simulink model "raspberrypi_MQTT_final"  (R2022b)
settings: Solver=FixedStepAuto  StartTime=0.0  StopTime=inf  RelTol=1e-3  EnableMultiTasking=on
undefined symbols (not defined in the file): hw
libraries: raspberrypiAVlib x1, raspberrypiIOTlib x1, dspspect3 x1, audiofilters x1, dspsigops x1
settings Model: Creator=The MathWorks, Inc.  LastModifiedBy=alex
settings SolverCC: AlgebraicLoopSolver=TrustRegion  PositivePriorityOrder=on  MaxZcPerStep=1
settings DataIOCC: ReturnWorkspaceOutputs=off
settings OptimizationCC: EnhancedBackFolding=on  PassReuseOutputArgsThreshold=0  MaxStackSize=64  OptimizeBlockOrder=speed  DifferentSizesBufferReuse=on  OptimizationCustomize=off
settings DebuggingCC: ParameterTunabilityLossMsg=error  UnconnectedInputMsg=warning  UnconnectedOutputMsg=warning  UnconnectedLineMsg=warning  PregeneratedLibrarySubsystemCodeDiagnostic=none  SFMachineParentedDataDiag=warning  ArithmeticOperatorsInVariantConditions=warning
settings HardwareCC: ProdBitPerPointer=32  ProdBitPerSizeT=32  ProdBitPerPtrDiffT=32  ProdLargestAtomicInteger=Long  ProdLargestAtomicFloat=Double  ProdWordSize=32  ProdHWDeviceType=ARM Compatible->ARM Cortex  UseEmbeddedCoderFeatures=off  UseSimulinkCoderFeatures=off
settings ModelReferenceCC: EnableRefExpFcnMdlSchedulingChecks=on
settings SFSimCC: SimUseLocalCustomCode=off  MATLABDynamicMemAlloc=off  CustomCodeUndefinedFunction=UseInterfaceOnly
settings RTWCC: Description=Embedded Coder  SystemTargetFile=ert.tlc  HardwareBoard=Raspberry Pi  TLCOptions="-aInlineSetEventsForThisBaseRateFcn=TLC_FALSE -aSuppressMultiTaskScheduler=TLC_FALSE  -aRateBasedStepFcn=0"  TemplateMakefile=ert_default_tmf  GenerateReport=on  RTWUseLocalCustomCode=off  Toolchain=GNU GCC Embedded Linux  BuildConfiguration=Faster Runs  LaunchReport=on  DLArmComputeVersion=19.05
settings CodeAppCC: ForceParamTrailComments=on  OperatorAnnotations=on
settings ERTTargetCC: ERTCustomFileBanners=off  SupportContinuousTime=on  SupportNonInlinedSFcns=on  RemoveResetFunc=off  SupportVariableSizeSignals=on  ModelStepFunctionPrototypeControlCompliant=off

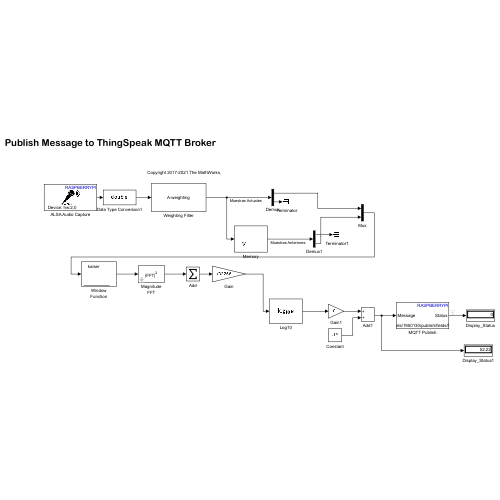
[thumbnail: Simulink's stored preview of the top-level diagram]
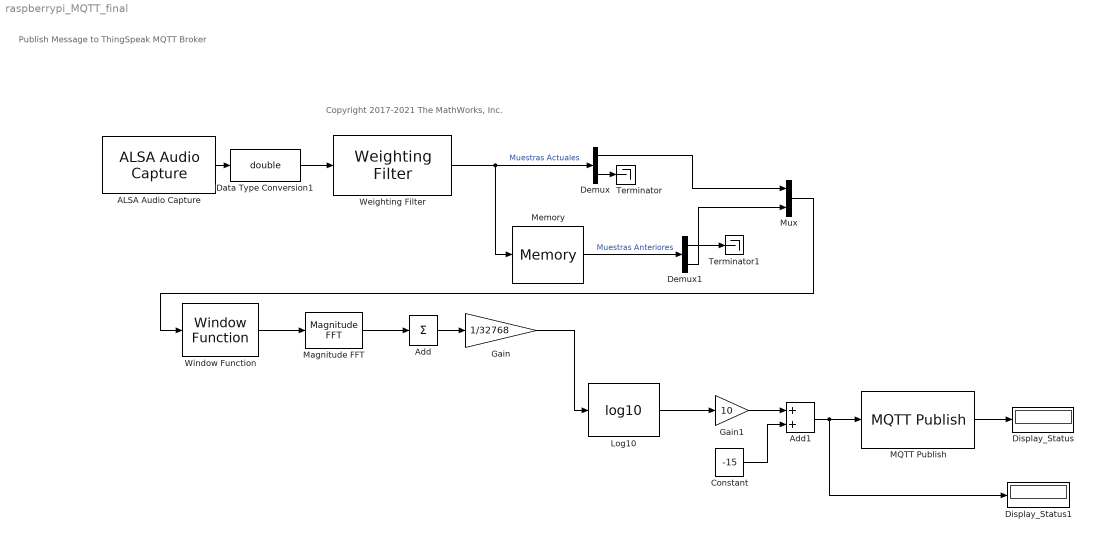
== system raspberrypi_MQTT_final ==
  note: Publish Message to ThingSpeak MQTT Broker
  note: Copyright 2017-2021 The MathWorks, Inc.
  ALSA Audio Capture : raspberrypiAVlib/ALSA Audio Capture  deviceStr=hw:2,0  DataBitDepth=16-bit integer  numberOfChannels=1  sampleRateEnum=44100  frameSize=22050  QueueDuration=0.5  blockPlatform=RASPBERRYPI
  Add : Sum  Inputs=+
  Add1 : Sum
  Constant : Constant  Value=-15
  Data Type Conversion1 : DataTypeConversion  OutDataTypeStr=double  RndMeth=Nearest
  Demux : Demux  Outputs=2
  Demux1 : Demux  Outputs=2
  Display_Status : Display
  Display_Status1 : Display
  Gain : Gain  Gain=1/32768
  Gain1 : Gain  Gain=10
  Log10 : Math  Operator=log10
  MQTT Publish : raspberrypiIOTlib/MQTT Publish  Topic=channels/1950130/publish/fields/field1  QoS=0  RetainMsg=off  blockPlatform=RASPBERRYPI
  Magnitude FFT : dspspect3/Magnitude FFT  mag_or_magsq=Magnitude squared  FFTImplementation=Auto  fftLenInherit=off  fftsize=32768  WrapInput=on
  Memory : Memory
  Mux : Mux  Inputs=2
  Terminator : Terminator
  Terminator1 : Terminator
  Weighting Filter : audiofilters/Weighting Filter  Method=A-weighting  InheritSampleRate=off  SampleRate=44100  SimulateUsing=Code generation  WorkspaceVariableName=myFilt  OverwriteExportVariable=on  MaskClassType=No mask
  Window Function : dspsigops/Window Function  winmode=Apply window to input  wintype=Kaiser  sampmode=Continuous  samptime=1  N=64  Rs=50  beta=5  winsamp=Symmetric  UserWindow=hamming  OptParams=off  UserParams={'symmetric'}  dataType=double  isSigned=on  wordLen=16  udDataType=sfix(16)  fracBitsMode=Best precision  numFracBits=15  roundingMode=Floor  overflowMode=off  numSidelobes=4  sidelobeLevel=-30
  wires:
  Data Type Conversion1/1 -> Weighting Filter/1
  Log10/1 -> Gain1/1
  Add/1 -> Gain/1
  Gain/1 -> Log10/1
  Magnitude FFT/1 -> Add/1
  Demux1/2 -> Mux/2
  Demux/2 -> Terminator/1
  Memory/1 -> Demux1/1  "Muestras Anteriores"
  Weighting Filter/1 -> Demux/1, Memory/1  "Muestras Actuales"
  Demux1/1 -> Terminator1/1
  Window Function/1 -> Magnitude FFT/1
  Constant/1 -> Add1/2
  Mux/1 -> Window Function/1
  Gain1/1 -> Add1/1
  Demux/1 -> Mux/1
  Add1/1 -> Display_Status1/1, MQTT Publish/1
  MQTT Publish/1 -> Display_Status/1
  ALSA Audio Capture/1 -> Data Type Conversion1/1
